simulink model "lidar_system_model"  (R2025b)
settings: Solver=FixedStepDiscrete  StartTime=0.0  StopTime=4e-5  FixedStep=5e-10  RelTol=1e-3
undefined symbols (not defined in the file or in its folder): magnitude
settings Model: Creator=Sarvik  LastModifiedBy=Sarvik

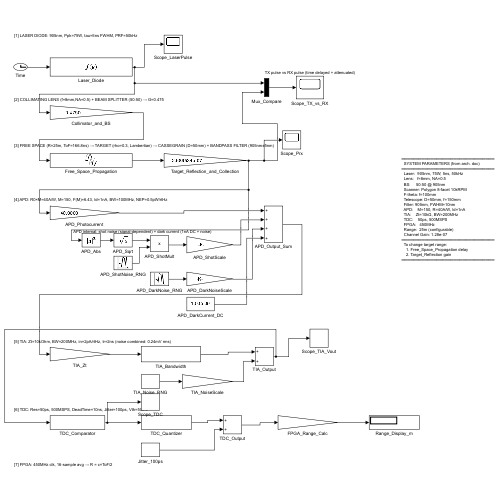
[thumbnail: Simulink's stored preview of the top-level diagram]
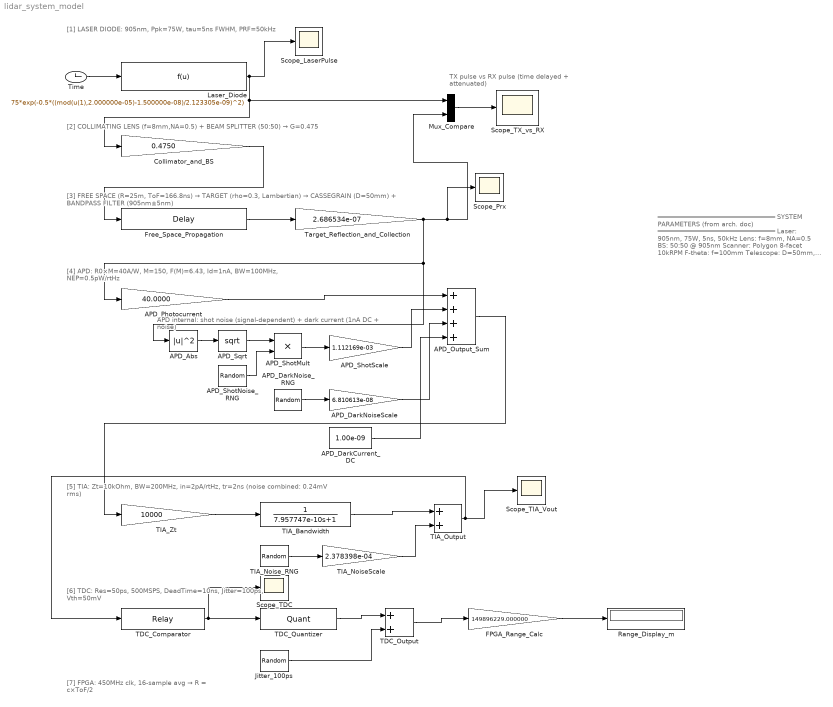
== system lidar_system_model ==
  note: [1] LASER DIODE: 905nm, Ppk=75W, tau=5ns FWHM, PRF=50kHz
  note: [2] COLLIMATING LENS (f=8mm,NA=0.5) + BEAM SPLITTER (50:50) → G=0.475
  note: [3] FREE SPACE (R=25m, ToF=166.8ns) → TARGET (rho=0.3, Lambertian) → CASSEGRAIN (D=50mm) + BANDPASS FILTER (905nm±5nm)
  note: [4] APD: R0×M=40A/W, M=150, F(M)=6.43, Id=1nA, BW=100MHz, NEP=0.5pW/rtHz
  note: APD internal: shot noise (signal-dependent) + dark current (1nA DC + noise)
  note: [5] TIA: Zt=10kOhm, BW=200MHz, in=2pA/rtHz, tr=2ns (noise combined: 0.24mV rms)
  note: [6] TDC: Res=50ps, 500MSPS, DeadTime=10ns, Jitter=100ps, Vth=50mV
  note: [7] FPGA: 450MHz clk, 16-sample avg → R = c×ToF/2
  note: TX pulse vs RX pulse (time delayed + attenuated)
  note: ════════════════════════════════
      |   SYSTEM PARAMETERS (from arch. doc)
      | ════════════════════════════════
      |   Laser:  905nm, 75W, 5ns, 50kHz
      |   Lens:   f=8mm, NA=0.5
      |   BS:     50:50 @ 905nm
      |   Scanner: Polygon 8-facet 10kRPM
      |   F-theta: f=100mm
      |   Telescope: D=50mm, f=150mm
      |   Filter: 905nm, FWHM=10nm
      |   APD:    M=150, R=40A/W, Id=1nA
      |   TIA:    Zt=10kΩ, BW=200MHz
      |   TDC:    50ps, 500MSPS
      |   FPGA:   450MHz
      |   Range:  25m (configurable)
      |   Channel Gain: 1.28e-07
      | ════════════════════════════════
      |   To change target range:
      |     1. Free_Space_Propagation delay
      |     2. Target_Reflection gain
      | ════════════════════════════════
  APD_Abs : Math  Operator=magnitude^2
  APD_DarkCurrent_DC : Constant  Value=1.00e-09
  APD_DarkNoiseScale : Gain  Gain=6.810613e-08
  APD_DarkNoise_RNG : RandomNumber  SampleTime=5e-10
  APD_Output_Sum : Sum  Inputs=++++
  APD_Photocurrent : Gain  Gain=40.0000
  APD_ShotMult : Product
  APD_ShotNoise_RNG : RandomNumber  SampleTime=5e-10
  APD_ShotScale : Gain  Gain=1.112169e-03
  APD_Sqrt : Math  Operator=sqrt
  Collimator_and_BS : Gain  Gain=0.4750
  FPGA_Range_Calc : Gain  Gain=149896229.000000
  Free_Space_Propagation : TransportDelay  DelayTime=1.6678204760e-07
  Jitter_100ps : RandomNumber  Variance=1.0000e-20  SampleTime=5e-10
  Laser_Diode : Fcn  Expr=75*exp(-0.5*((mod(u(1),2.000000e-05)-1.500000e-08)/2.123305e-09)^2)
  Mux_Compare : Mux  Inputs=2
  Range_Display_m : Display
  Scope_LaserPulse : Scope
  Scope_Prx : Scope
  Scope_TDC : Scope
  Scope_TIA_Vout : Scope
  Scope_TX_vs_RX : Scope
  TDC_Comparator : Relay  OnSwitchValue=0.0500  OffSwitchValue=0.0400
  TDC_Output : Sum
  TDC_Quantizer : Quantizer  QuantizationInterval=5.00e-11
  TIA_Bandwidth : TransferFcn  Denominator=[7.957747e-10 1]
  TIA_NoiseScale : Gain  Gain=2.378398e-04
  TIA_Noise_RNG : RandomNumber  SampleTime=5e-10
  TIA_Output : Sum
  TIA_Zt : Gain  Gain=10000
  Target_Reflection_and_Collection : Gain  Gain=2.686534e-07
  Time : Clock
  wires:
  Time/1 -> Laser_Diode/1
  Laser_Diode/1 -> Collimator_and_BS/1, Mux_Compare/1, Scope_LaserPulse/1
  Collimator_and_BS/1 -> Free_Space_Propagation/1
  Free_Space_Propagation/1 -> Target_Reflection_and_Collection/1
  Target_Reflection_and_Collection/1 -> Scope_Prx/1, Mux_Compare/2, APD_Photocurrent/1, APD_Abs/1
  APD_Abs/1 -> APD_Sqrt/1
  APD_Sqrt/1 -> APD_ShotMult/1
  APD_ShotNoise_RNG/1 -> APD_ShotMult/2
  APD_ShotMult/1 -> APD_ShotScale/1
  APD_DarkNoise_RNG/1 -> APD_DarkNoiseScale/1
  APD_Photocurrent/1 -> APD_Output_Sum/1
  APD_ShotScale/1 -> APD_Output_Sum/2
  APD_DarkNoiseScale/1 -> APD_Output_Sum/3
  APD_DarkCurrent_DC/1 -> APD_Output_Sum/4
  APD_Output_Sum/1 -> TIA_Zt/1
  TIA_Zt/1 -> TIA_Bandwidth/1
  TIA_Noise_RNG/1 -> TIA_NoiseScale/1
  TIA_Bandwidth/1 -> TIA_Output/1
  TIA_NoiseScale/1 -> TIA_Output/2
  TIA_Output/1 -> Scope_TIA_Vout/1, TDC_Comparator/1
  TDC_Comparator/1 -> TDC_Quantizer/1, Scope_TDC/1
  TDC_Quantizer/1 -> TDC_Output/1
  Jitter_100ps/1 -> TDC_Output/2
  TDC_Output/1 -> FPGA_Range_Calc/1
  FPGA_Range_Calc/1 -> Range_Display_m/1
  Mux_Compare/1 -> Scope_TX_vs_RX/1
